simulink model "F450_model_CA"  (R2022a)
settings: Solver=ode4  StartTime=0.0  StopTime=10  FixedStep=0.001  RelTol=1e-3
settings Model: Creator=ADMIN  LastModifiedBy=김응태
settings DebuggingCC: UnconnectedInputMsg=warning  UnconnectedOutputMsg=warning  UnconnectedLineMsg=warning
settings RTWCC: DLArmComputeVersion=19.05

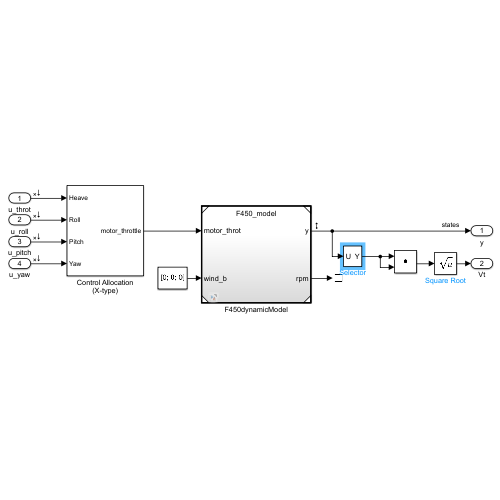
[thumbnail: Simulink's stored preview of the top-level diagram]
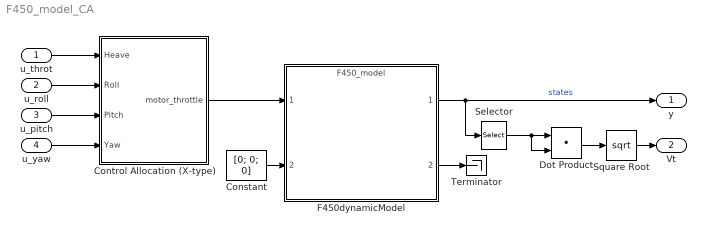
== system F450_model_CA ==
  u_throt : Inport
  u_roll : Inport  Port=2
  u_pitch : Inport  Port=3
  u_yaw : Inport  Port=4
  Constant : Constant  Value=[0; 0; 0]
  Control Allocation (X-type) : Subsystem
  Dot Product : DotProduct  OutDataTypeStr=Inherit: Inherit via internal rule
  F450dynamicModel : ModelReference  ModelNameDialog=F450_model.slx  SimulationMode=Normal  ModelReferenceVersion=10.81
  Selector : Selector  InputPortWidth=12  IndexOptions=Index vector (dialog)  Indices=[1 2 3]  OutputSizes=1
  Square Root : Sqrt
  Terminator : Terminator
  y : Outport
  Vt : Outport  Port=2
  wires:
  u_throt/1 -> Control Allocation (X-type)/1(Heave)
  F450dynamicModel/2 -> Terminator/1
  Control Allocation (X-type)/1(motor_throttle) -> F450dynamicModel/1
  F450dynamicModel/1 -> Selector/1, y/1  "states"
  u_pitch/1 -> Control Allocation (X-type)/3(Pitch)
  u_roll/1 -> Control Allocation (X-type)/2(Roll)
  u_yaw/1 -> Control Allocation (X-type)/4(Yaw)
  Constant/1 -> F450dynamicModel/2
  Dot Product/1 -> Square Root/1
  Square Root/1 -> Vt/1
  Selector/1 -> Dot Product/2, Dot Product/1

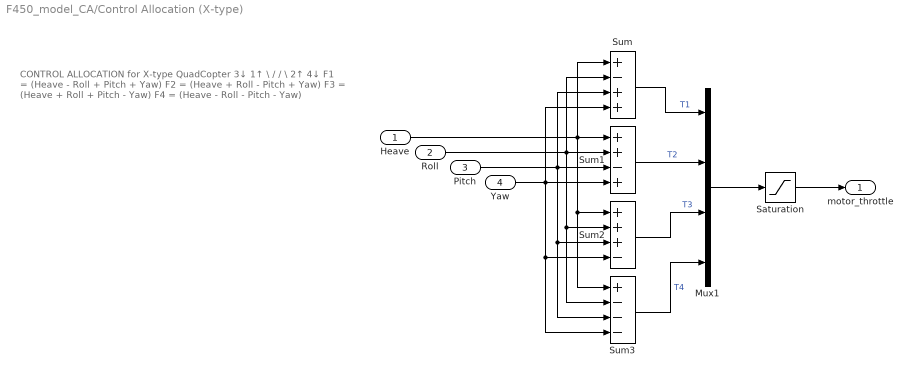
== system F450_model_CA/Control Allocation (X-type) ==
  note: CONTROL ALLOCATION for X-type QuadCopter
      | 3↓ 1↑
      | \ /
      | / \
      | 2↑ 4↓
      | F1 = (Heave - Roll + Pitch + Yaw)
      | F2 = (Heave + Roll - Pitch + Yaw)
      | F3 = (Heave + Roll + Pitch - Yaw)
      | F4 = (Heave - Roll - Pitch - Yaw)
  Heave : Inport
  Roll : Inport  Port=2
  Pitch : Inport  Port=3
  Yaw : Inport  Port=4
  Mux1 : Mux
  Saturation : Saturate  UpperLimit=1  LowerLimit=0
      settings: AttributesFormatString=%<LowerLimit>~%<UpperLimit>
  Sum : Sum  Inputs=+-++
  Sum1 : Sum  Inputs=++-+
  Sum2 : Sum  Inputs=+++-
  Sum3 : Sum  Inputs=+---
  motor_throttle : Outport
  wires:
  Sum2/1 -> Mux1/3  "T3"
  Sum/1 -> Mux1/1  "T1"
  Heave/1 -> Sum1/1, Sum/1, Sum2/1, Sum3/1
  Roll/1 -> Sum1/2, Sum/2, Sum2/2, Sum3/2
  Sum1/1 -> Mux1/2  "T2"
  Mux1/1 -> Saturation/1
  Sum3/1 -> Mux1/4  "T4"
  Pitch/1 -> Sum1/3, Sum/3, Sum2/3, Sum3/3
  Yaw/1 -> Sum1/4, Sum/4, Sum2/4, Sum3/4
  Saturation/1 -> motor_throttle/1
